simulink model "experiment_supervisor_user"  (R2023b)
settings: Solver=VariableStepDiscrete  StartTime=0.0  StopTime=inf  RelTol=1e-3
PreLoadFcn:
  | run('experiment_supervisor_data');
model workspace (MAT data in the model file):
  Ts = 0.01
undefined symbols (not defined in the file): current_target_timetable, ind, MCControlModes
libraries: dspswit3 x1, sldrtlib x1
settings Model: DataDictionary=amcbldc.sldd  SimulationMode=accelerator  Creator=mfussi  LastModifiedBy=mfussi
settings OptimizationCC: GainParamInheritBuiltInType=on  DefaultUnderspecifiedDataType=single  ReuseModelBlockBuffer=off  SimCompilerOptimization=on
settings DebuggingCC: UnconnectedInputMsg=warning  UnconnectedOutputMsg=warning  UnconnectedLineMsg=warning
settings HardwareCC: ProdBitPerLong=64  ProdHWDeviceType=Intel->x86-64 (Linux 64)
settings ModelReferenceCC: EnableRefExpFcnMdlSchedulingChecks=on
settings RTWCC: Description=Simulink Desktop Real-Time  SystemTargetFile=sldrt.tlc  TemplateMakefile=sldrt.tmf  TargetLang=C++  RTWCompilerOptimization=on  DLArmComputeVersion=19.05
settings CodeAppCC: MaxIdLength=95
settings SimulinkDesktopRealTimeCC: TargetLibSuffix=_sldrt.a  TargetPreCompLibLocation=C:\Program Files\MATLAB\R2023b\toolbox\sldrt\lib\win64  TargetLangStandard=C++11 (ISO)

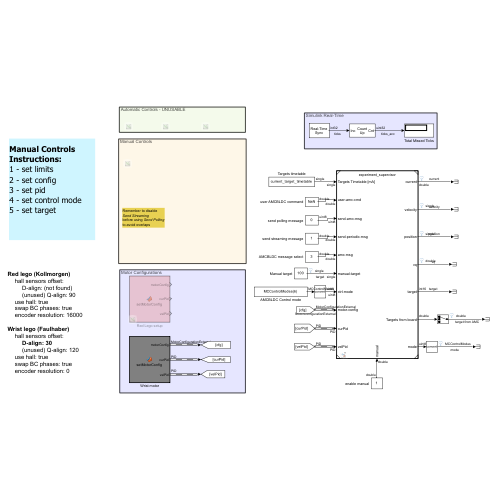
[thumbnail: Simulink's stored preview of the top-level diagram]
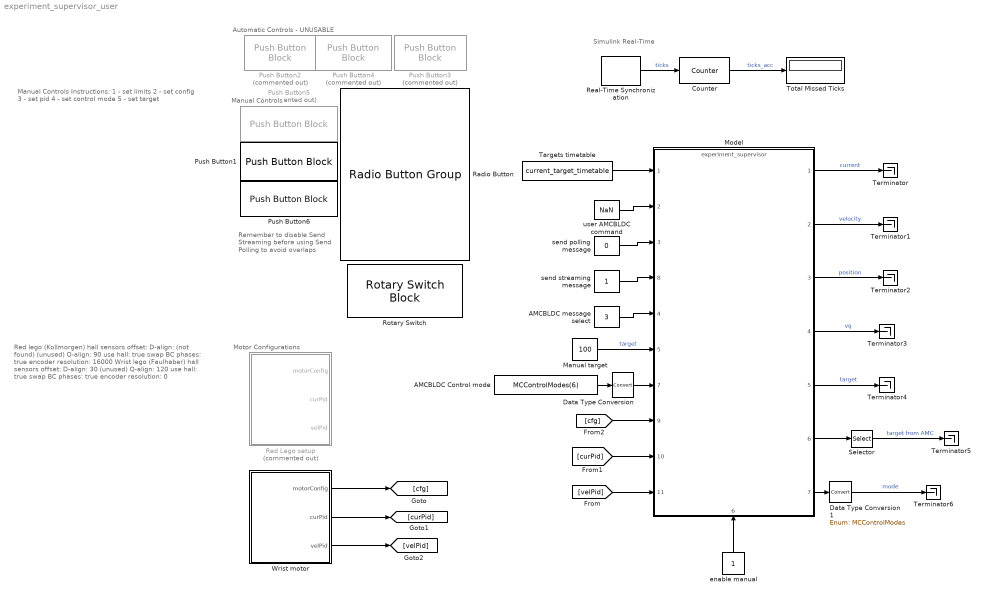
== system experiment_supervisor_user ==
  note: Manual Controls Instructions:
      | 1 - set limits
      | 2 - set config
      | 3 - set pid
      | 4 - set control mode
      | 5 - set target
  note: Motor Configurations
  note: Red lego (Kollmorgen)
      | hall sensors offset:
      | D-align: (not found)
      | (unused) Q-align: 90
      | use hall: true
      | swap BC phases: true
      | encoder resolution: 16000
      |
      | Wrist lego (Faulhaber)
      | hall sensors offset:
      | D-align: 30
      | (unused) Q-align: 120
      | use hall: true
      | swap BC phases: true
      | encoder resolution: 0
  note: Remember to disable
      | Send Streaming
      | before using Send Polling
      | to avoid overlaps
  note: Simulink Real-Time
  note: Manual Controls
  note: Automatic Controls - UNUSABLE
  AMCBLDC Control mode : Constant  Value=MCControlModes(6)
  AMCBLDC message select : Constant  Value=3
  Counter : dspswit3/Counter  Direction=Up  CountEvent=Rising edge  CounterSize=32 bits  MaxCount=255  InitialCount=0  Output=Count  HitValue=32  ResetInput=off  SamplesPerFrame=1  Ts=1  CntDtype=uint32  HitDtype=Logical
  Data Type Conversion : DataTypeConversion  SaturateOnIntegerOverflow=off  RndMeth=Floor
  Data Type Conversion1 : DataTypeConversion  OutDataTypeStr=Enum: MCControlModes  SaturateOnIntegerOverflow=off  RndMeth=Floor
  Manual target : Constant  Value=100  OutDataTypeStr=single
  Model : ModelReference  ModelNameDialog=experiment_supervisor.slx  SimulationMode=Normal  ModelReferenceVersion=5.38
      settings: PortSchema="{\"entries\":[{\"content\":{\"sides\":[{\"content\":{\"connectorIds\":[\"In1\",\"In2\",\"In3\",\"In8\",\"In4\",\"In5\",\"In7\",\"In9\",\"In10\",\"In11\"]},\"type\":\"ConnectorPlacement.EquallySpacedRectSide\",\"uuid\":\"82232601-ee00-4146-af62-83fa88e57da0\"},{\"content\":{\"connectorIds\":[\"Out1\",\"Out2\",\"Out3\",\"Out4\",\"Out5\",\"Out6\",\"Out7\"],\"side\":\"RIGHT\"},\"type\":\"ConnectorPlacement.EquallySpacedRectSide\",\"uuid\":\"78b9ecd1-2a7c-4f8d-9eb8-8deede0b59b2\"},{\"content\":{\"side\":\"TOP\"},\"type\":\"ConnectorPlacement.EquallySpacedRectSide\",\"uuid\":\"b60874bf-9c82-499b-91a1-b433f66db446\"},{\"content\":{\"connectorIds\":[\"In6\"],\"side\":\"BOTTOM\"},\"type\":\"ConnectorPlacement.EquallySpacedRectSide\",\"uuid\":\"63cf5cdc-0224-4041-8ff9-29fa2ef4ba12\"}]},\"type\":\"ConnectorPlacement.EquallySpacedConnector\",\"uuid\":\"7a4bae8c-d2ad-4163-94b1-1f3e0e1da4ed\"}],\"packageUris\":[\"http://schema.mathworks.com/mf0/Connector/R2020b\"],\"version\":\"1.0\"}"
  Push Button1 : PushButtonBlock  ButtonText=Send Polling CAN Msg  Icon=Triangle  IconAlignment=Right  IconColor=On  OffValue=0.000000
  Push Button2 : PushButtonBlock  Commented=on  ButtonText=Start  Icon=TurnSignalRight  IconAlignment=Right  IconColor=On  OffValue=-nan(ind)
  Push Button3 : PushButtonBlock  Commented=on  ButtonText=Reset  OnValue=2  Icon=Hexagon  IconAlignment=Right  IconColor=On  OffValue=2.000000
  Push Button4 : PushButtonBlock  Commented=on  ButtonText=Idle  OnValue=0  Icon=Circle  IconAlignment=Right  IconColor=On  OffValue=-1.000000
  Push Button5 : PushButtonBlock  Commented=on  ButtonText=Enable Manual Mode  ButtonType=Latch  IconAlignment=Right  OffValue=0.000000
  Push Button6 : PushButtonBlock  ButtonText=Send Streaming CAN Msg  ButtonType=Latch  Icon=TurnSignalRight  IconAlignment=Right  IconColor=On  OffValue=0.000000
  Radio Button : RadioButtonGroup  LabelPosition=Hide  SelectedLabel=set-target  ButtonGroupName=Manual CAN Messages
      settings: Values={{'set-control-mode-idle', 'set-control-mode', 'set-target', 'set-limits', 'discover', 'set-current-pid', 'set-velocity-pid', 'set-motor-config'}, [1 2 3 4 5 6 7 8]}
  Real-Time Synchronization : sldrtlib/Real-Time Synchronization  SampleTime=Ts  MaxMissedTicks=inf  ShowMissedTicks=on  YieldWhenWaiting=off
  Red Lego setup : MATLAB Function  Commented=on  TreatAsAtomicUnit=on
  Rotary Switch : RotarySwitchBlock  LabelPosition=Hide  EnumeratedDataType=MCControlModes
      settings: Values={{'Idle', 'OpenLoop', 'Velocity', 'Current'}, [0 80 10 6]}
  Selector : Selector  InputPortWidth=3  IndexOptions=Index vector (dialog)  Indices=[1]  OutputSizes=1
  Targets timetable : Constant  Value=current_target_timetable  OutDataTypeStr=single
  Terminator{,1..6} (7 alike) : Terminator
  Total Missed Ticks : Display
      settings: Decimation=5
  Wrist motor : MATLAB Function  TreatAsAtomicUnit=on
  enable manual : Constant
  send polling message : Constant  Value=0  OutDataTypeStr=uint8
  send streaming message : Constant
  user AMCBLDC command : Constant  Value=NaN
  wires:
  Targets timetable/1 -> Model/1
  user AMCBLDC command/1 -> Model/2
  AMCBLDC message select/1 -> Model/4
  Manual target/1 -> Model/5  "target"
  enable manual/1 -> Model/6
  Real-Time Synchronization/1 -> Counter/1  "ticks"
  Counter/1 -> Total Missed Ticks/1  "ticks_acc"
  Model/1 -> Terminator/1  "current"
  Model/4 -> Terminator3/1  "vq"
  Model/2 -> Terminator1/1  "velocity"
  Model/3 -> Terminator2/1  "position"
  Model/5 -> Terminator4/1  "target"
  AMCBLDC Control mode/1 -> Data Type Conversion/1
  send polling message/1 -> Model/3
  send streaming message/1 -> Model/8
  Data Type Conversion/1 -> Model/7
  Model/6 -> Selector/1
  Selector/1 -> Terminator5/1  "target from AMC"
  Wrist motor/1(motorConfig) -> [cfg]
  Wrist motor/2(curPid) -> [curPid]
  Wrist motor/3(velPid) -> [velPid]
  [velPid] -> Model/11
  [curPid] -> Model/10
  [cfg] -> Model/9
  Model/7 -> Data Type Conversion1/1
  Data Type Conversion1/1 -> Terminator6/1  "mode"

== matlab function experiment_supervisor_user/Red Lego setup ==
  data: motorConfig output Bus: MotorConfig; curPid output Bus: PIDConfig; velPid output Bus: PIDConfig
function [motorConfig, curPid, velPid] = setMotorConfig()

motorConfig.hall_sens_offset = single(30); % deg
motorConfig.has_hall_sens = true;
motorConfig.has_quadrature_encoder = true;
motorConfig.has_speed_quadrature_encoder = false;
motorConfig.has_torque_sens = false;
motorConfig.use_index = false;
motorConfig.enable_verbosity = true;
motorConfig.rotor_encoder_resolution = int16(16000);
motorConfig.rotor_index_offset = int16(0);
motorConfig.encoder_tolerance = uint8(0);
motorConfig.pole_pairs = uint8(4);
motorConfig.Kbemf = single(0);
motorConfig.Rphase = single(0);
motorConfig.Imin = single(-1e3);
motorConfig.Imax = single(1e3);
motorConfig.Vcc = single(24);
motorConfig.Vmax = single(24);

% Hall offset and BC phases swap is not available as a CAN message
% The parameters need to be changed in rtw_motor_config.c
swap_bc = 1;

% ---------------------------------

curPid.OutMax = single(100);
curPid.OutMin = single(-100);
curPid.P = single(2);
curPid.I = single(500);
curPid.D = single(0);
curPid.N = single(100);
curPid.I0 = single(0);
curPid.D0 = single(0);
curPid.shift_factor = uint8(0);


velPid.OutMax = single(1000);
velPid.OutMin = single(-1000);
velPid.P = single(1000);
velPid.I = single(1000);
velPid.D = single(0);
velPid.N = single(100);
velPid.I0 = single(0);
velPid.D0 = single(0);
velPid.shift_factor = uint8(10);

== matlab function experiment_supervisor_user/Wrist motor ==
  data: motorConfig output Bus: MotorConfigurationExternal; curPid output Bus: PID; velPid output Bus: PID
function [motorConfig, curPid, velPid] = setMotorConfig()


motorConfig.enable_verbosity = false;
motorConfig.has_hall_sens = true;
motorConfig.has_quadrature_encoder = false;
motorConfig.has_speed_quadrature_encoder = false;
motorConfig.has_torque_sens = false;
motorConfig.encoder_tolerance = uint8(0);
motorConfig.pole_pairs = uint8(7);
motorConfig.rotor_encoder_resolution = int16(0); % set to 0 to use only hall sensors
motorConfig.rotor_index_offset = int16(0);
motorConfig.use_index = false;


% motorConfig.Kbemf = single(0);
% motorConfig.Rphase = single(0);
% motorConfig.Imin = single(-1e3);
% motorConfig.Imax = single(1e3);
% motorConfig.Vmax = single(44);
% motorConfig.resistance = single(25.9);
% motorConfig.inductance = single(271);
% motorConfig.thermal_resistance = single(56);
% motorConfig.thermal_time_constant = single(270);

% Hall offset and BC phases swap is not available as a CAN message
% The parameters need to be changed in rtw_motor_config.c
swap_bc = 1;

% ---------------------------------

curPid.type = ControlModes.Current;
curPid.OutMax = single(100);
curPid.OutMin = single(-100);
curPid.P = single(2);
curPid.I = single(500);
curPid.D = single(0);
curPid.N = single(100);
curPid.I0 = single(0);
curPid.D0 = single(0);
curPid.shift_factor = uint8(0);

velPid.type = ControlModes.Velocity;
velPid.OutMax = single(1000);
velPid.OutMin = single(-1000);
velPid.P = single(-1000);
velPid.I = single(-1000);
velPid.D = single(0);
velPid.N = single(100);
velPid.I0 = single(0);
velPid.D0 = single(0);
velPid.shift_factor = uint8(10);
